simulink model "two_mass_model_1_R"  (R2021b)
settings: Solver=ode8  StartTime=0.0  StopTime=3  FixedStep=0.001  RelTol=1e-3
values from neighbouring files (symbols this model uses):
  C = 0.16    [compare_PRs.m]    (also in compare_steps.m; create_training_set.m; rbfnn_ts.mat; rbfnn_ts_4.mat)
  c0 = c_0*1    [calc_PR.m]    (also in rbfnn_ts.mat = 20.6001366722)
  c1 = c_1 + c_0*2*0.001    [calc_PR.m]    (also in rbfnn_ts.mat = 1.04120027334)
  C12 = C12_nom    [calc_params_sensivity.m]    (also in compare_PRs.m = C12*max(C12_v); compare_steps.m = C12*max(C12_v); create_training_set.m = C12_v(i); create_training_set_v2.m = 0.65)
  c2 = 2*0.001*c_1 + c_0*0.001^2    [calc_PR.m]    (also in rbfnn_ts.mat = 0.00202060013667)
  c3 = c_1*0.001^2    [calc_PR.m]    (also in rbfnn_ts.mat = 1e-06)
  J1 = J1_nom    [calc_params_sensivity.m]    (also in compare_PRs.m = J1*max(J1_v); compare_steps.m = J1*max(J1_v); create_training_set.m = J1_v(i); create_training_set_v2.m = 0.015)
  J2 = J2_nom    [calc_params_sensivity.m]    (also in compare_PRs.m = J2*max(J2_v); compare_steps.m = J2*max(J2_v); create_training_set.m = J2_v(i); create_training_set_v2.m = 0.05)
  Kd = Kd_v(i)    [calc_params_sensivity.m]    (also in compare_PRs.m = Kd*max(Kd_v); compare_steps.m = Kd*max(Kd_v); create_training_set.m; create_training_set_v2.m = 0.01)
  Ksp = 7    [compare_PRs.m]    (also in compare_steps.m; create_training_set.m; create_training_set_v2.m = 43.75; rbfnn_ts.mat)
  pref_gain = 10*(C*c0/Ksp + r0)    [calc_params_sensivity.m]    (also in compare_PRs.m = 10*(A0*c0 + B0*r0)/B0; compare_steps.m = 10*(A0*c0 + B0*r0)/B0; create_training_set.m; rbfnn_ts.mat = 95.8126802885)
  r0 = X(6,1)    [calc_PR.m]    (also in rbfnn_ts.mat = 9.11040776205)
  r1 = X(5,1)    [calc_PR.m]    (also in rbfnn_ts.mat = 1.38670293092)
  r2 = X(4,1)    [calc_PR.m]    (also in rbfnn_ts.mat = 0.695918527374)
  r3 = X(3,1)    [calc_PR.m]    (also in rbfnn_ts.mat = 0.0372641835349)
  Ra = 3.15    [compare_PRs.m]    (also in compare_steps.m; create_training_set.m; rbfnn_ts.mat; rbfnn_ts_4.mat)
  Ta = 0.05    [compare_PRs.m]    (also in compare_steps.m; create_training_set.m; rbfnn_ts.mat; rbfnn_ts_4.mat)
settings Model: Creator=Ilya  LastModifiedBy=Ilya

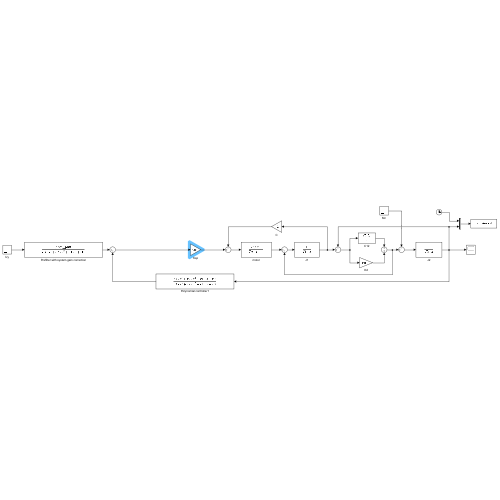
[thumbnail: Simulink's stored preview of the top-level diagram]
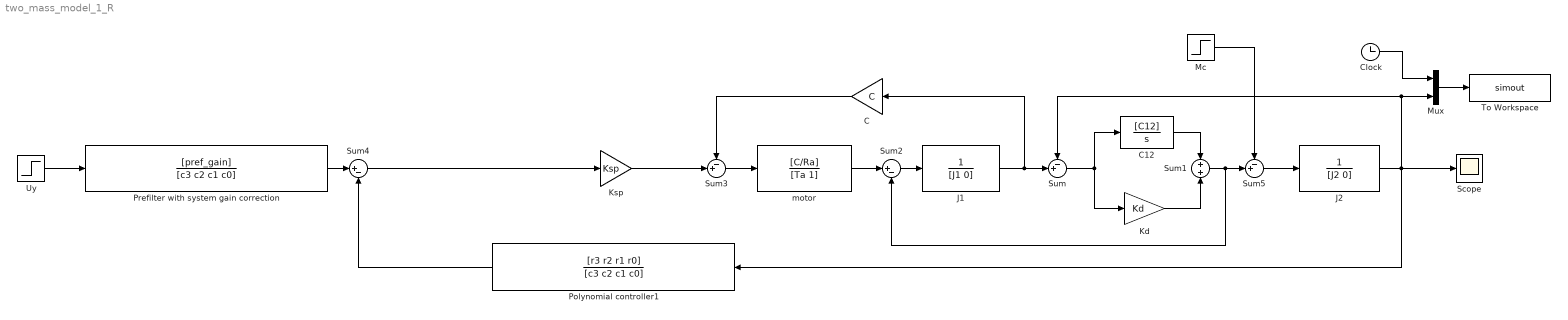
== system two_mass_model_1_R ==
  C : Gain  Gain=C
  C12 : TransferFcn  Numerator=[C12]  Denominator=[1 0]
  Clock : Clock
  J1 : TransferFcn  Denominator=[J1 0]
  J2 : TransferFcn  Denominator=[J2 0]
  Kd : Gain  Gain=Kd
  Ksp : Gain  Gain=Ksp
  Mc : Step  Time=3.01  After=0  SampleTime=0
  Mux : Mux  Inputs=2
  Polynomial controller1 : TransferFcn  Numerator=[r3 r2 r1 r0]  Denominator=[c3 c2 c1 c0]
  Prefilter with system gain correction : TransferFcn  Numerator=[pref_gain]  Denominator=[c3 c2 c1 c0]
  Scope : Scope
  Sum : Sum  Inputs=-+|
  Sum1 : Sum  Inputs=+|+
  Sum2 : Sum  Inputs=|+-
  Sum3 : Sum  Inputs=-+|
  Sum4 : Sum  Inputs=|+-
  Sum5 : Sum  Inputs=-+|
  To Workspace : ToWorkspace  VariableName=simout  SampleTime=-1
  Uy : Step  Time=0  After=10  SampleTime=0
  motor : TransferFcn  Numerator=[C/Ra]  Denominator=[Ta 1]
  wires:
  J1/1 -> C/1, Sum/2
  Sum/1 -> Kd/1, C12/1
  Kd/1 -> Sum1/2
  C12/1 -> Sum1/1
  Sum1/1 -> Sum5/2, Sum2/2
  Sum2/1 -> J1/1
  Sum3/1 -> motor/1
  motor/1 -> Sum2/1
  Ksp/1 -> Sum3/2
  J2/1 -> Scope/1, Polynomial controller1/1, Mux/2, Sum/1
  Uy/1 -> Prefilter with system gain correction/1
  Prefilter with system gain correction/1 -> Sum4/1
  Mux/1 -> To Workspace/1
  Clock/1 -> Mux/1
  Sum5/1 -> J2/1
  Mc/1 -> Sum5/1
  Sum4/1 -> Ksp/1
  C/1 -> Sum3/1
  Polynomial controller1/1 -> Sum4/2
